simulink model "drawWorks_withLookup"  (R2018b)
settings: Solver=ode3  StartTime=0.0  StopTime=inf  RelTol=1e-3
PreLoadFcn:
  | addpath('CAD_Files');
  | warning('off','sm:sli:setup:compile:LocalSolverNotSupported');
  | 
  | loadScale = 3;
  | load limitsLookup.mat;
InitFcn:
  | Ts = 10e-4;        % SPS/Overall Simulation time step
  | Tssc = 10*Ts;       % Simscape simulation time step
  | 
  | G = 10;
  | Rdrum = 0.25;
  | Np = 5;
  | m_topdrive = 1000;
  | m_drillstring = 22500;
  | Rpulley = Rdrum;
  | 
  | m = m_topdrive + m_drillstring;
  | 
  | % Top/Bottom Distance
  | xtop = 48*0.3048;
  | xbott = 0;
  | 
  | % Maximum Torque/Power of Drive
  | Tmax = 8000*1.36;
  | Pmax = 1500*746;
  | 
  | % Initial Conditions
  | v0 = 0; %m/s
  | x0 = 0; %m
  | 
  | % Gravity
  | g = 9.8;
values from neighbouring files (symbols this model uses):
  distLowering = [-48 -47 -46 -45 -44 -43 -42 -41 -40 -39 -38 -37 ... (130 elements, 1x130)]    [limitsLookup.mat]
  distRaising = [0 0.1 0.2 0.3 0.4 0.5 0.6 0.7 0.8 0.9 1 1.1 ... (139 elements, 1x139)]    [limitsLookup.mat]
  loadIn = [23500 46000 68500 91000 93250 95500 97750 100000 102250 104500 106750 109000 ... (71 elements, 1x71)]    [DrawworksLimitData.mat]    (also in limitsLookup.mat)
  spdLowering = [-1500 -1500 -1500 -1500 -1500 -1500 -1500 -1500 -1500 -1500 -1483.12408278 -1433.71794393 ... (9230 elements, 71x130)]    [limitsLookup.mat]
  spdRaising = [7.42375457692 0 0 0 0 0 0 0 0 0 0 0 ... (9869 elements, 71x139)]    [limitsLookup.mat]
undefined symbols (not defined in the file or in its folder): DiscIntNeverNeededParam, X, Y, Z
libraries: sm_lib x38, fl_lib x14, nesl_utility x11, powerlib x6, simulink x6, spsDrivesDcBusModel x1
(part 1 of 2)
settings Model: Creator=jlesage  LastModifiedBy=jlesage
settings DataIOCC: SaveOutput=off  SignalLogging=off  DSMLogging=off  SaveTime=off
settings ExplorerConfigSet: InternalSimMechanicsExplorerSettings="<ExplorerConfiguration><canonicalview>default</canonicalview><AnimationSetting><BasePlaybackSpeed>1.0</BasePlaybackSpeed><PlaybackSpeedFactor>256.0</PlaybackSpeedFactor></AnimationSetting><TilePanel><TileInfo><Tiles Columns=\"1\" Count=\"1\" Rows=\"1\"><Column Weight=\"1\"/><Row Weight=\"1\"/><Tile Height=\"1\" Width=\"1\" X=\"0\" Y=\"0\"/></Tiles></TileInfo><SceneInfo><SceneViewer><BGColor><R>0.60000002384185791</R><G>0.60000002384185791</G><B>0.60000002384185791</B></BGColor><Camera><DoPerspective>off</DoPerspective><Position><X>4.3364080211050684</X><Y>-7.69010096822353528</Y><Z>10.5874852236011314</Z></Position><Center><X>-0.0853470869668693233</X><Y>1.05957776856095531</Y><Z>8.89555922243923014</Z></Center><Up><X>-0.0863591017029704255</X><Y>0.146899309055797511</Y><Z>0.985374395116894397</Z></Up><ViewLimDist>1</ViewLimDist><YLim>13.1346250998977876</YLim><XLim>16.5774012824701131</XLim></Camera></SceneViewer></SceneInfo></TilePanel><MechEditorPanel><Cameras/><GfxPanelCameraMap/><VideoCreator><PlaybackSpeedRatio>1.0</PlaybackSpeedRatio><FrameRate>30</FrameRate><VideoFormat>Motion JPEG AVI</VideoFormat><FrameSize>auto</FrameSize></VideoCreator></MechEditorPanel></ExplorerConfiguration>"

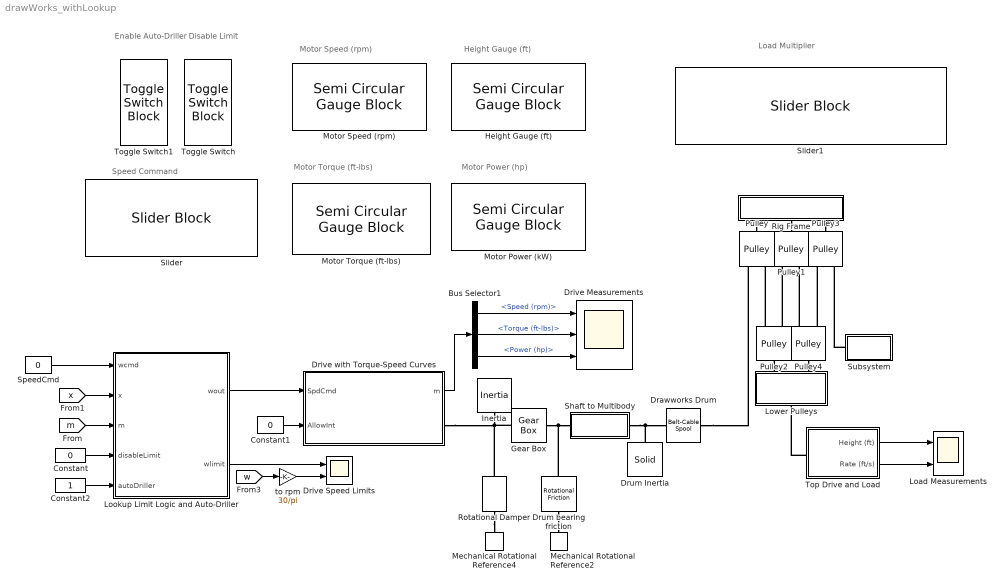
== system drawWorks_withLookup ==
  note: Height Gauge (ft)
  note: Motor Power (hp)
  note: Motor Torque (ft-lbs)
  note: Motor Speed (rpm)
  note: Load Multiplier
  note: Speed Command
  note: Disable
      | Limit
  note: Enable
      | Auto-Driller
  Bus Selector1 : BusSelector  OutputSignals=Mechanical.Speed (rpm),Mechanical.Torque (ft-lbs),Mechanical.Power (hp)
  Constant : Constant  Value=0  OutDataTypeStr=boolean
  Constant1 : Constant  Value=0
  Constant2 : Constant  OutDataTypeStr=boolean
  Drawworks Drum : sm_lib/Belts and Cables/Belt-Cable Spool  PitchRadius=Rdrum  PitchRadiusUnits=m  SenseSpoolAngleA=off  SenseFleetAngleA=off
      settings: SourceProductName=Simscape Multibody  SourceProductBaseCode=MS
  Drive Measurements : Scope  NumInputPorts=3
  Drive Speed Limits : Scope  NumInputPorts=2
  Drive with Torque-Speed Curves : Subsystem
  Drum Inertia : sm_lib/Body Elements/Solid  InertiaType=CalculateFromGeometry  Mass=0.01  MassUnits=kg  CenterOfMass=[0 0 0]  CenterOfMassUnits=m  MomentsOfInertia=[1 1 1]  MomentsOfInertiaUnits=kg*m^2  ProductsOfInertia=[0 0 0]  ProductsOfInertiaUnits=kg*m^2  BasedOnType=Density  Density=2700  DensityUnits=kg/m^3  DoExposeReferenceFrame=off  SerializedFrames=<Frames><Frame><Id>Frame1</Id><Value><Name>F1</Name><Origin><Source>ReferenceFrame</Source><FeatureName></FeatureName></Origin><PrimaryAxis><DefinedDirection>+Z</DefinedDirection><Source>ReferenceFrame</Source><SourceDirection>+Z</SourceDirection><FeatureName></FeatureName></PrimaryAxis><SecondaryAxis><DefinedDirection>+X</DefinedDirection><Source>ReferenceFrame</Source><SourceDirection>+X</SourceDirection><FeatureName></FeatureName></SecondaryAxis></Value></Frame></Frames>  GraphicType=FromGeometry  MarkerShape=Frame  MarkerSize=10  GraphicVisPropType=SimpleVisualProperties  GraphicDiffuseColor=[1.0 1.0 1.0]  GraphicSpecularColor=[0.8 0.8 0.8]  GraphicAmbientColor=[0.15 0.15 0.15 1.0]  GraphicEmissiveColor=[0.0 0.0 0.0 1.0]  GraphicShininess=10  GraphicOpacity=1.0  GeometryShape=Cylinder  RectangleSize=[1 1]  RectangleSizeUnits=m  BrickDimensions=[1 1 1]  BrickDimensionUnits=m  CylinderRadius=Rdrum  CylinderRadiusUnits=m  CylinderLength=0.75  CylinderLengthUnits=m  SphereRadius=0.5  SphereRadiusUnits=in  EllipsoidRadii=[1 1 1]*0.1  EllipsoidRadiiUnits=m  ExtrusionCrossSection=[1 1; -1 1; -1 -1; 1 -1]  ExtrusionCrossSectionUnits=m  ExtrusionLength=1  ExtrusionLengthUnits=m  PolygonNumSides=3  PolygonOuterRadius=1  PolygonOuterRadiusUnits=m  ExtGeomFileType=STEP  ExtGeomFileName=winch.step  ExtGeomFileUnits=m  RevolutionCrossSection=[1 1; 1 -1; 2 -1; 2 1]  RevolutionCrossSectionUnits=m  RevolutionExtent=Full  RevolutionAngle=180  RevolutionAngleUnits=deg
  Drum bearing friction : fl_lib/Mechanical/Rotational Elements/Rotational Friction  brkwy_trq=0.02*1.1 N*m  brkwy_vel=0.060623 rad/s  Col_trq=0.02 N*m  visc_coef=0.001 N*m/(rad/s)  w_specify=on  w_priority=Low  w=0 rad/s  w_nominal_specify=off  w_nominal_unit=rad/s  w_nominal_value=1  t_specify=off  t_priority=High  t=0 N*m  t_nominal_specify=off  t_nominal_unit=N*m  t_nominal_value=1
      settings: SourceProductName=Simscape
  Gear Box : fl_lib/Mechanical/Mechanisms/Gear Box  ratio=G  t_in_specify=off  t_in_priority=None  t_in=0 N*m  t_in_nominal_specify=off  t_in_nominal_unit=N*m  t_in_nominal_value=1  t_out_specify=off  t_out_priority=None  t_out=0 N*m  t_out_nominal_specify=off  t_out_nominal_unit=N*m  t_out_nominal_value=1
  Height Gauge (ft) : SemiCircularGaugeBlock  WebBlockId=1281  LabelPosition=Hide  ScaleMax=50  TickInterval=10
  Inertia : fl_lib/Mechanical/Rotational Elements/Inertia  inertia=0.01 kg*m^2  w_specify=off  w_priority=High  w=0 rad/s  w_nominal_specify=off  w_nominal_unit=rad/s  w_nominal_value=1  t_specify=off  t_priority=High  t=0 N*m  t_nominal_specify=off  t_nominal_unit=N*m  t_nominal_value=1
  Load Measurements : Scope  NumInputPorts=2
  Lookup Limit Logic and Auto-Driller : Stateflow chart  TreatAsAtomicUnit=on  SystemSampleTime=Tssc
  Lower Pulleys : Subsystem
  Mechanical Rotational Reference2 : fl_lib/Mechanical/Rotational Elements/Mechanical Rotational Reference
  Mechanical Rotational Reference4 : fl_lib/Mechanical/Rotational Elements/Mechanical Rotational Reference
  Motor Power (kW) : SemiCircularGaugeBlock  WebBlockId=1282  ScaleMin=-2000  ScaleMax=2000  TickInterval=1000
  Motor Speed (rpm) : SemiCircularGaugeBlock  WebBlockId=1283  ScaleMin=-1500  ScaleMax=1500  TickInterval=500
  Motor Torque (ft-lbs) : SemiCircularGaugeBlock  WebBlockId=1284  ScaleMin=-15000  ScaleMax=15000  TickInterval=5000
  Pulley{,1..4} (5 alike) : sm_lib/Belts and Cables/Pulley  PitchRadius=Rdrum  PitchRadiusUnits=m  SenseWrapAngle=off  SensePulleyAngleA=off  SensePulleyAngleB=off  SenseFleetAngleA=off  SenseFleetAngleB=off
      settings: SourceProductName=Simscape Multibody  SourceProductBaseCode=MS
  Rig Frame : Subsystem
  Rotational Damper : fl_lib/Mechanical/Rotational Elements/Rotational Damper  D=0.001 N*m/(rad/s)  w_specify=off  w_priority=High  w=0 rad/s  w_nominal_specify=off  w_nominal_unit=rad/s  w_nominal_value=1  t_specify=off  t_priority=High  t=0 N*m  t_nominal_specify=off  t_nominal_unit=N*m  t_nominal_value=1
  Shaft to Multibody : Subsystem
  Slider : SliderBlock  WebBlockId=1132  LabelPosition=Hide  ScaleMin=-1500  ScaleMax=1500
  Slider1 : SliderBlock  WebBlockId=1290  LabelPosition=Hide  ScaleMax=8  TickInterval=1
  SpeedCmd : Constant  Value=0  OutDataTypeStr=double
  Subsystem : Subsystem
  Toggle Switch : ToggleSwitchBlock  WebBlockId=1329  LabelPosition=Hide
      settings: Values={{'Off', 'On'}, [0 1]}
  Toggle Switch1 : ToggleSwitchBlock  WebBlockId=1330  LabelPosition=Hide
      settings: Values={{'Off', 'On'}, [0 1]}
  Top Drive and Load : Subsystem
  to rpm : Gain  Gain=30/pi
  wires:
  Bus Selector1/2 -> Drive Measurements/2  "<Torque (ft-lbs)>"
  Bus Selector1/3 -> Drive Measurements/3  "<Power (hp)>"
  Bus Selector1/1 -> Drive Measurements/1  "<Speed (rpm)>"
  [w] -> to rpm/1
  to rpm/1 -> Drive Speed Limits/2
  Constant1/1 -> Drive with Torque-Speed Curves/2(AllowInt)
  Drive with Torque-Speed Curves/1(m) -> Bus Selector1/1
  Top Drive and Load/1(Height (ft)) -> Load Measurements/1
  Top Drive and Load/2(Rate (ft/s)) -> Load Measurements/2
  SpeedCmd/1 -> Lookup Limit Logic and Auto-Driller/1(wcmd)
  [m] -> Lookup Limit Logic and Auto-Driller/3(m)
  [x] -> Lookup Limit Logic and Auto-Driller/2(x)
  Lookup Limit Logic and Auto-Driller/1(wout) -> Drive with Torque-Speed Curves/1(SpdCmd)
  Lookup Limit Logic and Auto-Driller/2(wlimit) -> Drive Speed Limits/1
  Constant2/1 -> Lookup Limit Logic and Auto-Driller/5(autoDriller)
  Constant/1 -> Lookup Limit Logic and Auto-Driller/4(disableLimit)
  connections:
  Drawworks Drum/RConn1 -- Pulley/RConn1
  Pulley4/RConn1 -- Pulley1/RConn2
  Pulley2/RConn1 -- Pulley/RConn2
  Subsystem/LConn1 -- Pulley3/RConn2
  Pulley4/RConn2 -- Pulley3/RConn1
  Pulley2/RConn2 -- Pulley1/RConn1
  Rig Frame/RConn1 -- Pulley/LConn1
  Rig Frame/RConn2 -- Pulley1/LConn1
  Rig Frame/RConn3 -- Pulley3/LConn1
  Lower Pulleys/RConn1 -- Pulley2/LConn1
  Pulley4/LConn1 -- Lower Pulleys/RConn2
  Drum Inertia/LConn1 -- Drawworks Drum/LConn1 -- Shaft to Multibody/RConn1
  Drum bearing friction/LConn1 -- Gear Box/RConn1 -- Shaft to Multibody/LConn1
  Drum bearing friction/RConn1 -- Mechanical Rotational Reference2/LConn1
  Rotational Damper/RConn1 -- Mechanical Rotational Reference4/LConn1
  Rotational Damper/LConn1 -- Gear Box/LConn1 -- Drive with Torque-Speed Curves/RConn1 -- Inertia/LConn1
  Top Drive and Load/LConn1 -- Lower Pulleys/LConn1

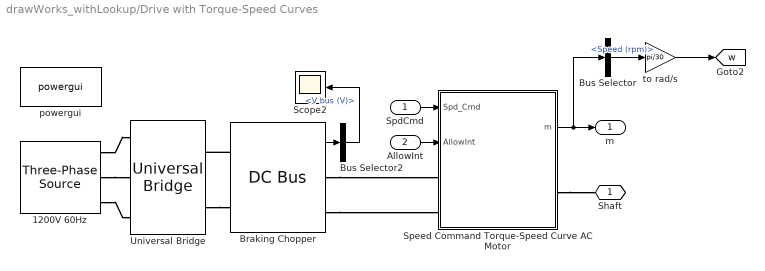
== system drawWorks_withLookup/Drive with Torque-Speed Curves ==
  SpdCmd : Inport
  AllowInt : Inport  Port=2
  1200V 60Hz : powerlib/Electrical Sources/Three-Phase Source  InternalConnection=Yg  VoltagePhases=off  Voltage=1200  PhaseAngle=0  Voltage_phases=[25e3 25e3 25e3]/sqrt(3)  PhaseAngles_phases=[0 -120 +120]  Frequency=60  NonIdealSource=off  SpecifyImpedance=on  Resistance=0.02  Inductance=0.05e-3  ShortCircuitLevel=500e6  BaseVoltage=5000  XRratio=7  BusType=swing  Pref=0  Qref=0  Prefabc=[10e3, 10e3, 10e3]  Qrefabc=[0, 0, 0]  Qmin=-inf  Qmax=inf
      settings: SourceProductName=Simscape Electrical
  Braking Chopper : spsDrivesDcBusModel/DC Bus   busType=Capacitive (generic)  Ts=Ts  capacitance=7500e-4  inductance=1e-3  Setx0=on  InitialVoltage=1000  Rbrake=8  frequency=500  activationVoltage=1200  shutdownVoltage=500
      settings: SourceProductName=The database C:\Users\ak23510\AppData\Roaming\MathWorks\MATLAB\R2017a\slblocks_master.db is locked, or a table in the database is locked. (database is locked)
  Bus Selector : BusSelector  OutputSignals=Mechanical.Speed (rpm)
  Bus Selector2 : BusSelector  OutputSignals=V bus (V)
  Scope2 : Scope
  Speed Command Torque-Speed Curve AC Motor : Subsystem  mask{contTrq=[10880,10880,10177,8905,7915,7124,6476,5699,4749,4071,3562], contSpd=[0 600 700 800 900 1000 1100 1250 1500 1750 2000], intTrq=[10880,10880,10177,8905,7915,7124,6476,5699,4749,4071,3562], intSpd=[0 600 700 800 900 1000 1100 1250 1500 1750 2000], intTime=1.5, offTime=7, Kp=15, Ki=1.5, wrate=750, Eff=99, T_alg=0.01}
      mask prompts: contTrq "Continuous Torque Limit (ft-lbs)"; contSpd "Continuous Speed Vector (rpm)"; intTrq "Intermittent Torque Limit (ft-lbs)"; intSpd "Intermittent Speed Vector (rpm)"; intTime "Time allowed above Steady-State (s)"; offTime "Cooldown Time (s)"; Kp "Speed Proportional Gain, Kp"; Ki "Speed Integral Gain, Ki"; wrate "Speed rate (rpm/s)"; Eff "Power Motor Efficiency (%)"; T_alg "Power Algebraic Loop Time Constant (s)"
      mask DialogControl Container4 Prompt: Torque-Speed Curves
      mask DialogControl Container6 Prompt: Controls
  Universal Bridge : powerlib/Power Electronics/Universal Bridge  Arms=3  SnubberResistance=1e5  SnubberCapacitance=inf  Device=Diodes  Ron=1e-3  Lon=0  ForwardVoltages="[  0  0  ]"  ForwardVoltage=0  GTOparameters=[ 10e-6 , 20e-6 ]  IGBTparameters=[ 1e-6 , 2e-6 ]  Measurements=All voltages and currents  Measurements_2=None  converterType=Rectifier
  powergui : powerlib/powergui  Priority=1  SimulationMode=Discrete  SampleTime=Ts  frequency=60  Iterations=50  frequencyindice=60  Pbase=100e6  ErrMax=1e-4  UnitsV=kV  UnitsW=MW  buscounter=0  FunctionMessages=off  echomessages=off  EnableUseOfTLC=off  CurrentSourceSwitches=off  DisableSnubberDevices=off  DisableRonSwitches=off  DisableVfSwitches=off  DisplayEquations=off  SolverType=Tustin/Backward Euler (TBE)  Interpol=off  ExternalGateDelay=off  methode=off  Ts=100  x0status=blocks  SPID=on  SwTol=0  HookPort=off  RestoreLinks=warning  ResistiveCurrentMeasurement=off  Frange=[0:2:500]  Ylog=off  Xlog=on  ShowGrid=off  save=off  variable=ZData  structure=0  ZoomFFT=off  StartTime=0.0  cycles=1  DisplayStyle=1  fundamental=60  FreqAxis=off  MaxFrequency=1000  frequencyindicesteady=1  RmsSteady=1  display=off
  to rad/s : Gain  Gain=pi/30
  Shaft : PMIOPort  Side=Right
  m : Outport
  tag scope: w=global
  wires:
  Braking Chopper/1 -> Bus Selector2/1
  Bus Selector2/1 -> Scope2/1  "<V bus (V)>"
  SpdCmd/1 -> Speed Command Torque-Speed Curve AC Motor/1(Spd_Cmd)
  AllowInt/1 -> Speed Command Torque-Speed Curve AC Motor/2(AllowInt)
  Speed Command Torque-Speed Curve AC Motor/1(m) -> Bus Selector/1, m/1
  to rad/s/1 -> [w]
  Bus Selector/1 -> to rad/s/1  "<Speed (rpm)>"
  connections:
  1200V 60Hz/RConn3 -- Universal Bridge/LConn3
  1200V 60Hz/RConn2 -- Universal Bridge/LConn2
  Braking Chopper/RConn2 -- Speed Command Torque-Speed Curve AC Motor/LConn2
  Braking Chopper/RConn1 -- Speed Command Torque-Speed Curve AC Motor/LConn1
  1200V 60Hz/RConn1 -- Universal Bridge/LConn1
  Braking Chopper/LConn1 -- Universal Bridge/RConn1
  Universal Bridge/RConn2 -- Braking Chopper/LConn2
  Speed Command Torque-Speed Curve AC Motor/RConn1 -- Shaft/RConn1

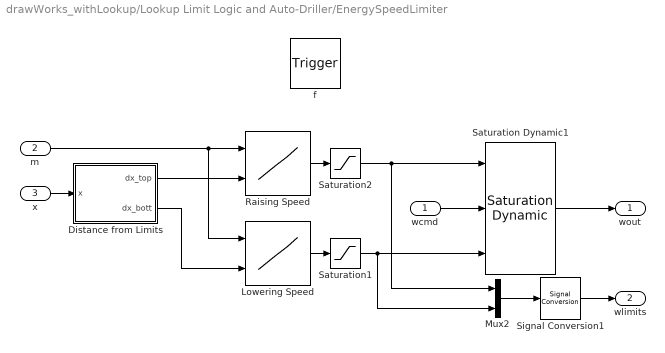
== system drawWorks_withLookup/Lookup Limit Logic and Auto-Driller/EnergySpeedLimiter ==
  wcmd : Inport  OutDataTypeStr=double  PortDimensions=1
  m : Inport  Port=2  OutDataTypeStr=double  PortDimensions=1
  x : Inport  Port=3  OutDataTypeStr=double  PortDimensions=1
  f : TriggerPort  TriggerType=function-call  VariantControl=(inherit)
      settings: CopyFcn=Stateflow.SLINSF.SimulinkMan.removeBlockPreDeleteFcn  PreDeleteFcn=Stateflow.SLINSF.SimulinkMan.unsafePredeleteFcn
  Distance from Limits : Subsystem
  Lowering Speed : Lookup_n-D  BreakpointsForDimension1=loadIn  BreakpointsForDimension2=distLowering  Table=spdLowering  InternalRulePriority=Speed  RndMeth=Simplest  InputSameDT=on
  Mux2 : Mux  Inputs=2
  Raising Speed : Lookup_n-D  BreakpointsForDimension1=loadIn  BreakpointsForDimension2=distRaising  Table=spdRaising  InternalRulePriority=Speed  RndMeth=Simplest  InputSameDT=on
  Saturation Dynamic1 : simulink/Discontinuities/Saturation Dynamic  OutMin=[]  OutMax=[]  OutDataTypeStr=Inherit: Same as second input  OutDataType=fixdt(1, 16)  OutScaling=2^-10  DoSatur=off
  Saturation1 : Saturate  UpperLimit=0  LowerLimit=-inf
  Saturation2 : Saturate  UpperLimit=inf  LowerLimit=0
  Signal Conversion1 : SignalConversion  OverrideOpt=off
  wout : Outport
  wlimits : Outport  Port=2
  wires:
  x/1 -> Distance from Limits/1(x)
  Saturation Dynamic1/1 -> wout/1
  Mux2/1 -> Signal Conversion1/1
  m/1 -> Lowering Speed/1, Raising Speed/1
  wcmd/1 -> Saturation Dynamic1/2
  Distance from Limits/2(dx_bott) -> Lowering Speed/2
  Distance from Limits/1(dx_top) -> Raising Speed/2
  Saturation1/1 -> Mux2/2, Saturation Dynamic1/3
  Lowering Speed/1 -> Saturation1/1
  Raising Speed/1 -> Saturation2/1
  Saturation2/1 -> Mux2/1, Saturation Dynamic1/1
  Signal Conversion1/1 -> wlimits/1

== system drawWorks_withLookup/Lower Pulleys ==
  Pulley 1 : Subsystem  mask{bottOffset=0.1}
      mask prompts: bottOffset "Bottom Offset"
  Pulley 2 : Subsystem  mask{bottOffset=-0.1}
      mask prompts: bottOffset "Bottom Offset"
  Load : PMIOPort  Side=Left
  P1 : PMIOPort  Port=2  Side=Right
  P2 : PMIOPort  Port=3  Side=Right
  connections:
  Pulley 1/LConn1 -- Pulley 2/LConn1 -- Load/RConn1
  Pulley 2/RConn1 -- P2/RConn1
  Pulley 1/RConn1 -- P1/RConn1

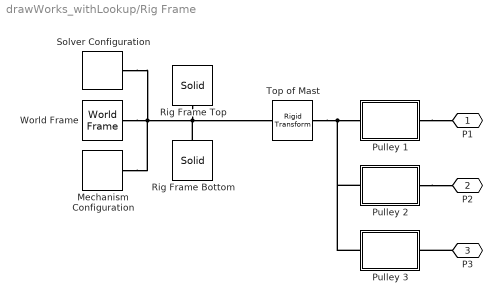
== system drawWorks_withLookup/Rig Frame ==
  Mechanism Configuration : sm_lib/Utilities/Mechanism Configuration  UniformGravity=Constant  GravityVector=[0 0 -9.80665]  GravityUnits=m/s^2  LinearizationDelta=0.001
  Pulley 1 : Subsystem  mask{topOffset=0.2}
      mask prompts: topOffset "Top Position [m]"
  Pulley 2 : Subsystem  mask{topOffset=0}
      mask prompts: topOffset "Top Position [m]"
  Pulley 3 : Subsystem  mask{topOffset=-0.2}
      mask prompts: topOffset "Top Position [m]"
  Rig Frame Top : sm_lib/Body Elements/Solid  InertiaType=CalculateFromGeometry  Mass=0.01  MassUnits=kg  CenterOfMass=[0 0 0]  CenterOfMassUnits=m  MomentsOfInertia=[1 1 1]  MomentsOfInertiaUnits=kg*m^2  ProductsOfInertia=[0 0 0]  ProductsOfInertiaUnits=kg*m^2  BasedOnType=Density  Density=2700  DensityUnits=kg/m^3  DoExposeReferenceFrame=off  SerializedFrames=<Frames><Frame><Id>Frame1</Id><Value><Name>F1</Name><Origin><Source>ReferenceFrame</Source><FeatureName></FeatureName></Origin><PrimaryAxis><DefinedDirection>+Z</DefinedDirection><Source>ReferenceFrame</Source><SourceDirection>+Y</SourceDirection><FeatureName></FeatureName></PrimaryAxis><SecondaryAxis><DefinedDirection>+X</DefinedDirection><Source>ReferenceFrame</Source><SourceDirection>+X</SourceDirection><FeatureName></FeatureName></SecondaryAxis></Value></Frame></Frames>  GraphicType=FromGeometry  MarkerShape=Frame  MarkerSize=10  GraphicVisPropType=SimpleVisualProperties  GraphicDiffuseColor=[1.0 0.0 0.2]  GraphicSpecularColor=[0.8 0.8 0.8]  GraphicAmbientColor=[0.15 0.15 0.15 1.0]  GraphicEmissiveColor=[0.0 0.0 0.0 1.0]  GraphicShininess=10  GraphicOpacity=1.0  GeometryShape=FromFile  RectangleSize=[1 1]  RectangleSizeUnits=m  BrickDimensions=[1 1 1]  BrickDimensionUnits=m  CylinderRadius=0.25  CylinderRadiusUnits=in  CylinderLength=1  CylinderLengthUnits=in  SphereRadius=0.5  SphereRadiusUnits=in  EllipsoidRadii=[1 1 1]*0.1  EllipsoidRadiiUnits=m  ExtrusionCrossSection=[1 1; -1 1; -1 -1; 1 -1]  ExtrusionCrossSectionUnits=m  ExtrusionLength=1  ExtrusionLengthUnits=m  PolygonNumSides=3  PolygonOuterRadius=1  PolygonOuterRadiusUnits=m  ExtGeomFileType=STEP  ExtGeomFileName=\CAD_Files\RigFrame_Top.STEP  ExtGeomFileUnits=m  RevolutionCrossSection=[1 1; 1 -1; 2 -1; 2 1]  RevolutionCrossSectionUnits=m  RevolutionExtent=Full  RevolutionAngle=180  RevolutionAngleUnits=deg
  Rig Frame Bottom : sm_lib/Body Elements/Solid  InertiaType=CalculateFromGeometry  Mass=0.01  MassUnits=kg  CenterOfMass=[0 0 0]  CenterOfMassUnits=m  MomentsOfInertia=[1 1 1]  MomentsOfInertiaUnits=kg*m^2  ProductsOfInertia=[0 0 0]  ProductsOfInertiaUnits=kg*m^2  BasedOnType=Density  Density=2700  DensityUnits=kg/m^3  DoExposeReferenceFrame=off  SerializedFrames=<Frames><Frame><Id>Frame1</Id><Value><Name>F1</Name><Origin><Source>ReferenceFrame</Source><FeatureName></FeatureName></Origin><PrimaryAxis><DefinedDirection>+Z</DefinedDirection><Source>ReferenceFrame</Source><SourceDirection>+Y</SourceDirection><FeatureName></FeatureName></PrimaryAxis><SecondaryAxis><DefinedDirection>+X</DefinedDirection><Source>ReferenceFrame</Source><SourceDirection>+X</SourceDirection><FeatureName></FeatureName></SecondaryAxis></Value></Frame></Frames>  GraphicType=FromGeometry  MarkerShape=Frame  MarkerSize=10  GraphicVisPropType=SimpleVisualProperties  GraphicDiffuseColor=[1.0 1.0 1.0]  GraphicSpecularColor=[0.8 0.8 0.8]  GraphicAmbientColor=[0.15 0.15 0.15 1.0]  GraphicEmissiveColor=[0.0 0.0 0.0 1.0]  GraphicShininess=10  GraphicOpacity=1.0  GeometryShape=FromFile  RectangleSize=[1 1]  RectangleSizeUnits=m  BrickDimensions=[1 1 1]  BrickDimensionUnits=m  CylinderRadius=0.25  CylinderRadiusUnits=in  CylinderLength=1  CylinderLengthUnits=in  SphereRadius=0.5  SphereRadiusUnits=in  EllipsoidRadii=[1 1 1]*0.1  EllipsoidRadiiUnits=m  ExtrusionCrossSection=[1 1; -1 1; -1 -1; 1 -1]  ExtrusionCrossSectionUnits=m  ExtrusionLength=1  ExtrusionLengthUnits=m  PolygonNumSides=3  PolygonOuterRadius=1  PolygonOuterRadiusUnits=m  ExtGeomFileType=STEP  ExtGeomFileName=\CAD_Files\RigFrame_Bottom.STEP  ExtGeomFileUnits=m  RevolutionCrossSection=[1 1; 1 -1; 2 -1; 2 1]  RevolutionCrossSectionUnits=m  RevolutionExtent=Full  RevolutionAngle=180  RevolutionAngleUnits=deg
  "Solver Configuration " : nesl_utility/Solver Configuration  PhysicalDomain=network_engine_domain  SubClassName=solver  LeftPortType=input  RightPortType=generic  Tones=[]  Harmonics=[]  SimulateNoise=off  Profile=off  UseLocalSampling=off  EnableSwitchedLinearOptims=on  FrequencyDomain=off  UseCCode=off  RelTol=0.001  AbsTol=1e-06  MinStep=1e-09  ToWorkspace=off  RevertToSquareIcSolve=off  NumHomotopyIterations=100  PhasorMode=off  PhasorModeNumHarmonics=1  DoDC=off  ResidualTolerance=1e-09  UseLocalSolver=on  LocalSolverChoice=NE_BACKWARD_EULER_ADVANCER  LocalSolverSampleTime=Tssc  DoFixedCost=on  MaxNonlinIter=3  MaxModeIter=2  LinearAlgebra=Sparse  EquationFormulation=NE_TIME_EF  DelaysMemoryBudget=1024  AutomaticFiltering=on  FilteringTimeConstant=0.001  PartitionStorageMethod=AS_NEEDED  PartitionMemoryBudget=1024
  Top of Mast : sm_lib/Frames and Transforms/Rigid Transform  TranslationMethod=Cartesian  TranslationStandardOffset=57.5  TranslationLengthUnit=ft  TranslationStandardAxis=+Z  TranslationCartesianOffset=[0 0 57.5]  TranslationROffset=0  TranslationROffsetUnits=m  TranslationZOffset=0  TranslationZOffsetUnits=m  TranslationThetaOffset=0  TranslationThetaOffsetUnits=deg  RotationMethod=StandardAxis  RotationAngleUnits=deg  RotationStandardAxis=+Y  RotationAngle=90  RotationArbitraryAxis=[0 0 1]  FollAlignAxisA=+X  BaseAlignAxisA=+Y  FollAlignAxisB=+Y  BaseAlignAxisB=+Z  RotationSequenceAxes=FollowerAxes  RotationSequence=XYX  RotationSequenceAngles=[0 0 0]  RotationSequenceAnglesUnits=deg  RotationMatrix=[1 0 0; 0 1 0; 0 0 1]
  World Frame : sm_lib/Frames and Transforms/World Frame
  P1 : PMIOPort  Side=Right
  P2 : PMIOPort  Port=2  Side=Right
  P3 : PMIOPort  Port=3  Side=Right
  connections:
  Top of Mast/RConn1 -- Pulley 3/LConn1 -- Pulley 2/LConn1 -- Pulley 1/LConn1
  Mechanism Configuration/RConn1 -- "Solver Configuration "/RConn1 -- World Frame/RConn1 -- Top of Mast/LConn1 -- Rig Frame Top/LConn1 -- Rig Frame Bottom/LConn1
  Pulley 1/RConn1 -- P1/RConn1
  P3/RConn1 -- Pulley 3/RConn1
  Pulley 2/RConn1 -- P2/RConn1

== system drawWorks_withLookup/Shaft to Multibody ==
  Drum Position : sm_lib/Frames and Transforms/Rigid Transform  TranslationMethod=Cartesian  TranslationStandardOffset=10  TranslationLengthUnit=ft  TranslationStandardAxis=+Y  TranslationCartesianOffset=[5 10 0]  TranslationROffset=0  TranslationROffsetUnits=m  TranslationZOffset=0  TranslationZOffsetUnits=m  TranslationThetaOffset=0  TranslationThetaOffsetUnits=deg  RotationMethod=StandardAxis  RotationAngleUnits=deg  RotationStandardAxis=-Y  RotationAngle=90  RotationArbitraryAxis=[0 0 1]  FollAlignAxisA=+X  BaseAlignAxisA=+Y  FollAlignAxisB=+Y  BaseAlignAxisB=+Z  RotationSequenceAxes=FollowerAxes  RotationSequence=XYX  RotationSequenceAngles=[0 0 0]  RotationSequenceAnglesUnits=deg  RotationMatrix=[1 0 0; 0 1 0; 0 0 1]
  Revolute Joint for Drum : sm_lib/Joints/Revolute Joint  SenseConstraintForce=off  SenseConstraintForceX=off  SenseConstraintForceY=off  SenseConstraintForceZ=off  SenseConstraintTorque=off  SenseConstraintTorqueX=off  SenseConstraintTorqueY=off  SenseConstraintTorqueZ=off  SenseTotalForce=off  SenseTotalForceX=off  SenseTotalForceY=off  SenseTotalForceZ=off  SenseTotalTorque=off  SenseTotalTorqueX=off  SenseTotalTorqueY=off  SenseTotalTorqueZ=off  CompositeWrenchDir=FollowerOnBase  CompositeWrenchFrame=BaseFrame  EquilibriumPosition=0  EquilibriumPositionUnits=deg  SpringStiffness=0  SpringStiffnessUnits=N*m/deg  DampingCoefficient=0  DampingCoefficientUnits=N*m/(deg/s)  TorqueActuationMode=InputTorque  MotionActuationMode=ComputedMotion  SensePosition=off  SenseVelocity=on  SenseAcceleration=off  SenseTorqueForce=off  PositionTargetSpecify=off  PositionTargetPriority=High  PositionTargetValue=0  PositionTargetValueUnits=deg  VelocityTargetSpecify=off  VelocityTargetPriority=High  VelocityTargetValue=0  VelocityTargetValueUnits=deg/s
  Rotational Simscape Intf : Subsystem
  World Frame2 : sm_lib/Frames and Transforms/World Frame
  Drum : PMIOPort  Side=Right
  Shaft : PMIOPort  Port=2  Side=Left
  connections:
  Drum Position/RConn1 -- Revolute Joint for Drum/LConn1
  Revolute Joint for Drum/RConn1 -- Drum/RConn1
  Rotational Simscape Intf/RConn1 -- Revolute Joint for Drum/LConn2
  World Frame2/RConn1 -- Drum Position/LConn1
  Shaft/RConn1 -- Rotational Simscape Intf/RConn2
  Rotational Simscape Intf/LConn1 -- Revolute Joint for Drum/RConn2

== system drawWorks_withLookup/Subsystem ==
  Anchor Position : sm_lib/Frames and Transforms/Rigid Transform  TranslationMethod=Cartesian  TranslationStandardOffset=10  TranslationLengthUnit=ft  TranslationStandardAxis=+Y  TranslationCartesianOffset=[-5 10+Rdrum*3.2808 0]  TranslationROffset=0  TranslationROffsetUnits=m  TranslationZOffset=0  TranslationZOffsetUnits=m  TranslationThetaOffset=0  TranslationThetaOffsetUnits=deg  RotationMethod=StandardAxis  RotationAngleUnits=deg  RotationStandardAxis=-Y  RotationAngle=90  RotationArbitraryAxis=[0 0 1]  FollAlignAxisA=+X  BaseAlignAxisA=+Y  FollAlignAxisB=+Y  BaseAlignAxisB=+Z  RotationSequenceAxes=FollowerAxes  RotationSequence=XYX  RotationSequenceAngles=[0 0 0]  RotationSequenceAnglesUnits=deg  RotationMatrix=[1 0 0; 0 1 0; 0 0 1]
  Belt-Cable Properties : sm_lib/Belts and Cables/Belt-Cable Properties  DrumBeltCableAlignment=Unrestricted  GraphicType=PitchLine  GraphicVisPropType=SimpleVisualProperties  GraphicDiffuseColor=[0.0 0.0 0.0]  GraphicSpecularColor=[0.5 0.5 0.5 1.0]  GraphicAmbientColor=[0.15 0.15 0.15 1.0]  GraphicEmissiveColor=[0.0 0.0 0.0 1.0]  GraphicShininess=75  GraphicOpacity=1.0
      settings: SourceProductName=Simscape Multibody  SourceProductBaseCode=MS
  Belt-Cable End : sm_lib/Belts and Cables/Belt-Cable End
      settings: SourceProductName=Simscape Multibody  SourceProductBaseCode=MS
  World Frame3 : sm_lib/Frames and Transforms/World Frame
  Anchor : PMIOPort  Side=Left
  connections:
  World Frame3/RConn1 -- Anchor Position/LConn1
  Anchor Position/RConn1 -- Belt-Cable End/LConn1
  Belt-Cable End/RConn1 -- Anchor/RConn1 -- Belt-Cable Properties/LConn1

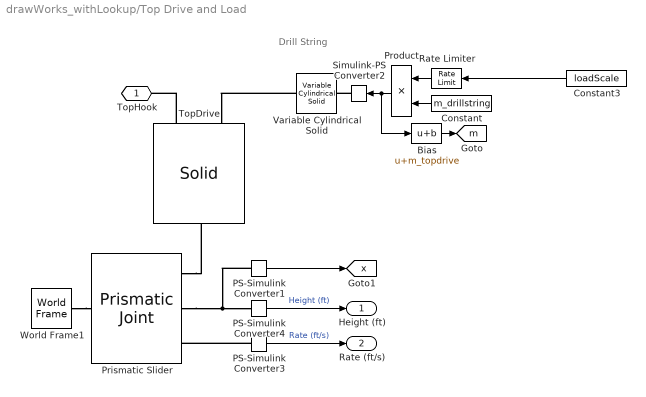
== system drawWorks_withLookup/Top Drive and Load ==
  note: Drill String
  Bias : Bias  Bias=m_topdrive
  Constant : Constant  Value=m_drillstring
  Constant3 : Constant  Value=loadScale
  PS-Simulink Converter1 : nesl_utility/PS-Simulink Converter  PhysicalDomain=network_engine_domain  SubClassName=ps_output  LeftPortType=input  RightPortType=output  PseudoPeriodic=off  Frequencies=[]  Unit=ft  AffineConversion=off
  PS-Simulink Converter3 : nesl_utility/PS-Simulink Converter  PhysicalDomain=network_engine_domain  SubClassName=ps_output  LeftPortType=input  RightPortType=output  PseudoPeriodic=off  Frequencies=[]  Unit=ft/s  AffineConversion=off
  PS-Simulink Converter4 : nesl_utility/PS-Simulink Converter  PhysicalDomain=network_engine_domain  SubClassName=ps_output  LeftPortType=input  RightPortType=output  PseudoPeriodic=off  Frequencies=[]  Unit=ft  AffineConversion=off
  Prismatic Slider : sm_lib/Joints/Prismatic Joint  SenseConstraintForce=off  SenseConstraintForceX=off  SenseConstraintForceY=off  SenseConstraintForceZ=off  SenseConstraintTorque=off  SenseConstraintTorqueX=off  SenseConstraintTorqueY=off  SenseConstraintTorqueZ=off  SenseTotalForce=off  SenseTotalForceX=off  SenseTotalForceY=off  SenseTotalForceZ=off  SenseTotalTorque=off  SenseTotalTorqueX=off  SenseTotalTorqueY=off  SenseTotalTorqueZ=off  CompositeWrenchDir=FollowerOnBase  CompositeWrenchFrame=BaseFrame  EquilibriumPosition=0  EquilibriumPositionUnits=m  SpringStiffness=0  SpringStiffnessUnits=N/m  DampingCoefficient=0  DampingCoefficientUnits=N/(m/s)  TorqueActuationMode=NoTorque  MotionActuationMode=ComputedMotion  SensePosition=on  SenseVelocity=on  SenseAcceleration=off  SenseTorqueForce=off  PositionTargetSpecify=off  PositionTargetPriority=High  PositionTargetValue=5  PositionTargetValueUnits=ft  VelocityTargetSpecify=off  VelocityTargetPriority=High  VelocityTargetValue=0  VelocityTargetValueUnits=m/s
  Product : Product
  Rate Limiter : RateLimiter  RisingSlewLimit=0.5  FallingSlewLimit=-0.5  SampleTimeMode=inherited  InitialCondition=loadScale
  Simulink-PS Converter2 : nesl_utility/Simulink-PS Converter  PhysicalDomain=network_engine_domain  SubClassName=ps_input  LeftPortType=input  RightPortType=output  PseudoPeriodic=off  Frequencies=[]  NoiseDistribution=none  NoiseParameters=[]  Unit=kg  AffineConversion=off  FilteringAndDerivatives=provide  SimscapeFilterOrder=1  InputFilterTimeConstant=0.001  UdotUserProvided=0
  TopDrive : sm_lib/Body Elements/Solid  InertiaType=PointMass  Mass=m_topdrive  MassUnits=kg  CenterOfMass=[0 0 0]  CenterOfMassUnits=m  MomentsOfInertia=[1 1 1]  MomentsOfInertiaUnits=kg*m^2  ProductsOfInertia=[0 0 0]  ProductsOfInertiaUnits=kg*m^2  BasedOnType=Density  Density=1000  DensityUnits=kg/m^3  DoExposeReferenceFrame=off  SerializedFrames=<Frames><Frame><Id>Frame1</Id><Value><Name>TopHook</Name><Origin><Source>GeometricFeature</Source><FeatureName>cylindrical surface 11</FeatureName></Origin><PrimaryAxis><DefinedDirection>+Z</DefinedDirection><Source>ReferenceFrame</Source><SourceDirection>+Y</SourceDirection><FeatureName></FeatureName></PrimaryAxis><SecondaryAxis><DefinedDirection>+X</DefinedDirection><Source>ReferenceFrame</Source><SourceDirection>+X</SourceDirection><FeatureName></FeatureName></SecondaryAxis></Value></Frame><Frame><Id>Frame2</Id><Value><Name>COM</Name><Origin><Source>GeometricFeature</Source><FeatureName>planar surface 22</FeatureName></Origin><PrimaryAxis><DefinedDirection>+Z</DefinedDirection><Source>ReferenceFrame</Source><SourceDirection>+Y</SourceDirection><FeatureName></FeatureName></PrimaryAxis><SecondaryAxis><DefinedDirection>+X</DefinedDirection><Source>ReferenceFrame</Source><SourceDirection>+X</SourceDirection><FeatureName></FeatureName></SecondaryAxis></Value></Frame><Frame><Id>Frame3</Id><Value><Name>String</Name><Origin><Source>GeometricFeature</Source><FeatureName>planar surface 23</FeatureName></Origin><PrimaryAxis><DefinedDirection>+Z</DefinedDirection><Source>ReferenceFrame</Source><SourceDirection>-Y</SourceDirection><FeatureName></FeatureName></PrimaryAxis><SecondaryAxis><DefinedDirection>+X</DefinedDirection><Source>ReferenceFrame</Source><SourceDirection>+X</SourceDirection><FeatureName></FeatureName></SecondaryAxis></Value></Frame></Frames>  GraphicType=FromGeometry  MarkerShape=Sphere  MarkerSize=10  GraphicVisPropType=SimpleVisualProperties  GraphicDiffuseColor=[0.8 0.8 0.0]  GraphicSpecularColor=[0.5 0.5 0.5 1.0]  GraphicAmbientColor=[0.15 0.15 0.15 1.0]  GraphicEmissiveColor=[0.0 0.0 0.0 1.0]  GraphicShininess=75  GraphicOpacity=1.0  GeometryShape=FromFile  RectangleSize=[1 1]  RectangleSizeUnits=m  BrickDimensions=[1 1 1]*4  BrickDimensionUnits=in  CylinderRadius=1  CylinderRadiusUnits=m  CylinderLength=1  CylinderLengthUnits=m  SphereRadius=1  SphereRadiusUnits=m  EllipsoidRadii=[1 1 1]  EllipsoidRadiiUnits=m  ExtrusionCrossSection=[1 1; -1 1; -1 -1; 1 -1]  ExtrusionCrossSectionUnits=m  ExtrusionLength=1  ExtrusionLengthUnits=m  PolygonNumSides=3  PolygonOuterRadius=1  PolygonOuterRadiusUnits=m  ExtGeomFileType=STEP  ExtGeomFileName=\CAD_Files\TopDrive.STEP  ExtGeomFileUnits=m  RevolutionCrossSection=[1 1; 1 -1; 2 -1; 2 1]  RevolutionCrossSectionUnits=m  RevolutionExtent=Full  RevolutionAngle=180  RevolutionAngleUnits=deg
  Variable Cylindrical Solid : sm_lib/Body Elements/Variable Mass/Variable Cylindrical Solid  LengthType=CalculateFromMass  Length=1  LengthUnits=m  RadiusType=Constant  Radius=0.1  RadiusUnits=m  MassType=ProvidedByInput  InitialMassType=Specified  InitialMass=1  InitialMassUnits=kg  Density=1000  DensityUnits=kg/m^3  SenseRadius=off  SenseLength=off  SenseMass=off  SenseCenterOfMass=off  SenseInertiaMatrix=off  GraphicType=Marker  MarkerShape=Cube  MarkerSize=10  GraphicVisPropType=SimpleVisualProperties  GraphicDiffuseColor=[0.5 0.5 0.5]  GraphicSpecularColor=[0.5 0.5 0.5 1.0]  GraphicAmbientColor=[0.15 0.15 0.15 1.0]  GraphicEmissiveColor=[0.0 0.0 0.0 1.0]  GraphicShininess=75  GraphicOpacity=1.0
      settings: SourceProductName=Simscape Multibody  SourceProductBaseCode=MS
  World Frame1 : sm_lib/Frames and Transforms/World Frame
  TopHook : PMIOPort  Side=Left
  Height (ft) : Outport
  Rate (ft/s) : Outport  Port=2
  tag scope: m=global, x=global
  wires:
  PS-Simulink Converter1/1 -> [x]
  Constant/1 -> Product/2
  Bias/1 -> [m]
  Constant3/1 -> Rate Limiter/1
  Product/1 -> Bias/1, Simulink-PS Converter2/1
  PS-Simulink Converter4/1 -> Height (ft)/1  "Height (ft)"
  PS-Simulink Converter3/1 -> Rate (ft/s)/1  "Rate (ft/s)"
  Rate Limiter/1 -> Product/1
  connections:
  Prismatic Slider/RConn2 -- PS-Simulink Converter1/LConn1 -- PS-Simulink Converter4/LConn1
  Prismatic Slider/RConn1 -- TopDrive/RConn1
  Simulink-PS Converter2/RConn1 -- Variable Cylindrical Solid/LConn1
  Variable Cylindrical Solid/RConn1 -- TopDrive/LConn2
  World Frame1/RConn1 -- Prismatic Slider/LConn1
  PS-Simulink Converter3/LConn1 -- Prismatic Slider/RConn3
  TopDrive/LConn1 -- TopHook/RConn1

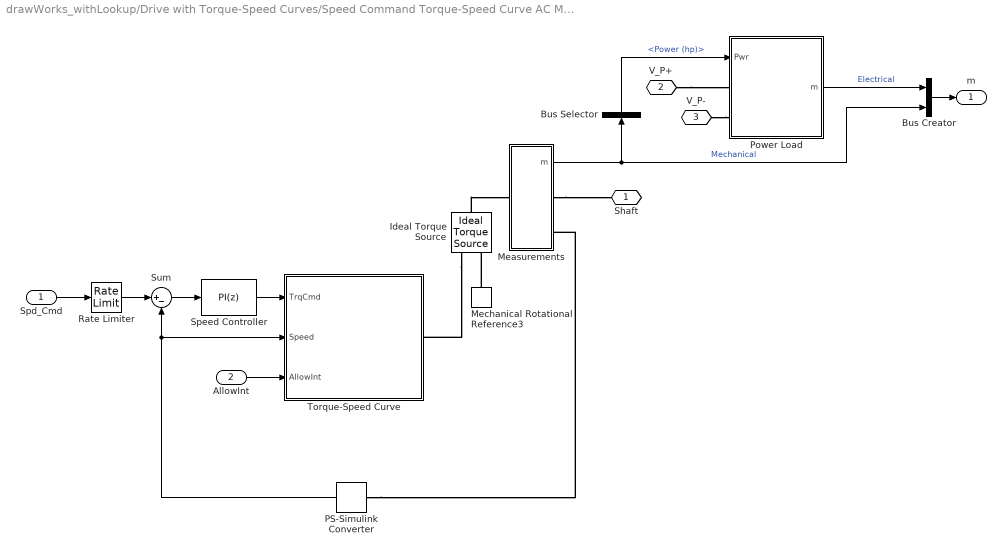
== system drawWorks_withLookup/Drive with Torque-Speed Curves/Speed Command Torque-Speed Curve AC Motor ==
  Spd_Cmd : Inport
  AllowInt : Inport  Port=2
  Bus Creator : BusCreator  Inputs=2
  Bus Selector : BusSelector  OutputSignals=Power (hp)
  Ideal Torque Source : fl_lib/Mechanical/Mechanical Sources/Ideal Torque Source
  Measurements : Subsystem
  Mechanical Rotational Reference3 : fl_lib/Mechanical/Rotational Elements/Mechanical Rotational Reference
  PS-Simulink Converter : nesl_utility/PS-Simulink Converter  PhysicalDomain=network_engine_domain  SubClassName=ps_output  LeftPortType=input  RightPortType=output  PseudoPeriodic=off  Frequencies=[]  Unit=rpm  AffineConversion=off
  Power Load : Subsystem  VariantControl=Variant
  Rate Limiter : RateLimiter  RisingSlewLimit=wrate  FallingSlewLimit=-wrate  SampleTimeMode=inherited
  Speed Controller : simulink/Continuous/PID Controller  Controller=PI  Form=Parallel  TimeDomain=Discrete-time  SampleTime=-1  IntegratorMethod=Forward Euler  FilterMethod=Forward Euler  ControllerParametersSource=internal  P=Kp  I=Ki  D=-9.19425038888835  UseFilter=on  N=3.08252405545653  TunerSelectOption=Transfer Function Based (PID Tuner App)  ZeroCross=off  InitialConditionSource=internal  InitialConditionForIntegrator=Rdrum/(G*(Np-1))*(m_topdrive+m_drillstring)*9.81*0.737562*loadScale  InitialConditionForFilter=0  DifferentiatorICPrevScaledInput=0  ExternalReset=none  TrackingMode=off  Kt=1  LimitOutput=on  UpperSaturationLimit=intTrq(1)  LowerSaturationLimit=-intTrq(1)  LinearizeAsGain=on  AntiWindupMode=clamping  Kb=1000  POutMin=[]  POutMax=[]  IOutMin=[]  IOutMax=[]  DOutMin=[]  DOutMax=[]  NOutMin=[]  NOutMax=[]  SumOutMin=[]  SumOutMax=[]  SaturationOutMin=[]  SaturationOutMax=[]  PParamMin=[]  PParamMax=[]  IParamMin=[]  IParamMax=[]  DParamMin=[]  DParamMax=[]  NParamMin=[]  NParamMax=[]  KbParamMin=[]  KbParamMax=[]  KtParamMin=[]  KtParamMax=[]  KbOutMin=[]  KbOutMax=[]  KtOutMin=[]  KtOutMax=[]  IntegratorOutMin=[]  IntegratorOutMax=[]  FilterOutMin=[]  FilterOutMax=[]  SumI1OutMin=[]  SumI1OutMax=[]  SumI2OutMin=[]  SumI2OutMax=[]  SumI3OutMin=[]  SumI3OutMax=[]  SumI4OutMin=[]  SumI4OutMax=[]  SumDOutMin=[]  SumDOutMax=[]  DifferentiatorOutMin=[]  DifferentiatorOutMax=[]  FilterDiffOutCoefMin=[]  FilterDiffOutCoefMax=[]  ReciprocalOutMin=[]  ReciprocalOutMax=[]  SumDenOutMin=[]  SumDenOutMax=[]  SumNumOutMin=[]  SumNumOutMax=[]  DivideOutMin=[]  DivideOutMax=[]  IntegratorContinuousStateAttributes=''  IntegratorStateMustResolveToSignalObject=off  IntegratorRTWStateStorageClass=Auto  FilterContinuousStateAttributes=''  FilterStateMustResolveToSignalObject=off  FilterRTWStateStorageClass=Auto  ParallelPVariant=InternalParameters  IdealPVariant=Disabled  IVariant=InternalParameters  DVariant=Disabled  IntegratorVariant=Discrete  SatVariant=Enabled  AWVariant=DiscClampingParallel  PCopyVariant=Disabled  TRVariant=Disabled  FdbkBlocksVariant=Forward  IdealPFdbkVariant=Disabled  SatFdbkVariant=Disabled  DerivativeFilterVariant=Disabled  NVariant=Disabled  NCopyVariant=Disabled_SignalSpec  FilterICVariant=Disabled  IntegratorICVariant=InternalICs  ExternalResetVariant=Disabled  TRSumVariant=Passthrough  SumFdbkVariant=Disabled  SumVariant=Sum_PI
  Sum : Sum  Inputs=|+-
  Torque-Speed Curve : Subsystem
  Shaft : PMIOPort  Side=Right
  V_P+ : PMIOPort  Port=2  Side=Left
  V_P- : PMIOPort  Port=3  Side=Left
  m : Outport
  wires:
  Measurements/1(m) -> Bus Selector/1, Bus Creator/2  "Mechanical"
  Rate Limiter/1 -> Sum/1
  Sum/1 -> Speed Controller/1
  Speed Controller/1 -> Torque-Speed Curve/1(TrqCmd)
  AllowInt/1 -> Torque-Speed Curve/3(AllowInt)
  PS-Simulink Converter/1 -> Sum/2, Torque-Speed Curve/2(Speed)
  Spd_Cmd/1 -> Rate Limiter/1
  Bus Selector/1 -> Power Load/1(Pwr)  "<Power (hp)>"
  Bus Creator/1 -> m/1
  Power Load/1(m) -> Bus Creator/1  "Electrical"
  connections:
  Mechanical Rotational Reference3/LConn1 -- Ideal Torque Source/RConn2
  Ideal Torque Source/LConn1 -- Measurements/LConn1
  PS-Simulink Converter/LConn1 -- Measurements/RConn2
  Measurements/RConn1 -- Shaft/RConn1
  Ideal Torque Source/RConn1 -- Torque-Speed Curve/RConn1
  V_P-/RConn1 -- Power Load/LConn2
  V_P+/RConn1 -- Power Load/LConn1

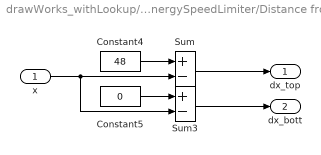
== system drawWorks_withLookup/Lookup Limit Logic and Auto-Driller/EnergySpeedLimiter/Distance from Limits ==
  x : Inport
  Constant4 : Constant  Value=48
  Constant5 : Constant  Value=0
  Sum : Sum  Inputs=+-
  Sum3 : Sum  Inputs=+-
  dx_top : Outport
  dx_bott : Outport  Port=2
  wires:
  Constant4/1 -> Sum/1
  Constant5/1 -> Sum3/1
  x/1 -> Sum/2, Sum3/2
  Sum/1 -> dx_top/1
  Sum3/1 -> dx_bott/1

== system drawWorks_withLookup/Lower Pulleys/Pulley 1 ==
  Offset from Load : sm_lib/Frames and Transforms/Rigid Transform  TranslationMethod=Cartesian  TranslationStandardOffset=57.5  TranslationLengthUnit=m  TranslationStandardAxis=+Z  TranslationCartesianOffset=[bottOffset 0 0]  TranslationROffset=0  TranslationROffsetUnits=m  TranslationZOffset=0  TranslationZOffsetUnits=m  TranslationThetaOffset=0  TranslationThetaOffsetUnits=deg  RotationMethod=StandardAxis  RotationAngleUnits=deg  RotationStandardAxis=+Y  RotationAngle=90  RotationArbitraryAxis=[0 0 1]  FollAlignAxisA=+X  BaseAlignAxisA=+Y  FollAlignAxisB=+Y  BaseAlignAxisB=+Z  RotationSequenceAxes=FollowerAxes  RotationSequence=XYX  RotationSequenceAngles=[0 0 0]  RotationSequenceAnglesUnits=deg  RotationMatrix=[1 0 0; 0 1 0; 0 0 1]
  Pulley Inertia : sm_lib/Body Elements/Solid  InertiaType=CalculateFromGeometry  Mass=0.01  MassUnits=kg  CenterOfMass=[0 0 0]  CenterOfMassUnits=m  MomentsOfInertia=[1 1 1]  MomentsOfInertiaUnits=kg*m^2  ProductsOfInertia=[0 0 0]  ProductsOfInertiaUnits=kg*m^2  BasedOnType=Density  Density=2700  DensityUnits=kg/m^3  DoExposeReferenceFrame=off  SerializedFrames=<Frames><Frame><Id>Frame1</Id><Value><Name>F1</Name><Origin><Source>GeometricFeature</Source><FeatureName>top surface</FeatureName></Origin><PrimaryAxis><DefinedDirection>+Z</DefinedDirection><Source>ReferenceFrame</Source><SourceDirection>+Z</SourceDirection><FeatureName></FeatureName></PrimaryAxis><SecondaryAxis><DefinedDirection>+X</DefinedDirection><Source>ReferenceFrame</Source><SourceDirection>+X</SourceDirection><FeatureName></FeatureName></SecondaryAxis></Value></Frame></Frames>  GraphicType=FromGeometry  MarkerShape=Frame  MarkerSize=10  GraphicVisPropType=SimpleVisualProperties  GraphicDiffuseColor=[1.0 1.0 1.0]  GraphicSpecularColor=[0.8 0.8 0.8]  GraphicAmbientColor=[0.15 0.15 0.15 1.0]  GraphicEmissiveColor=[0.0 0.0 0.0 1.0]  GraphicShininess=10  GraphicOpacity=1.0  GeometryShape=Cylinder  RectangleSize=[1 1]  RectangleSizeUnits=m  BrickDimensions=[1 1 1]  BrickDimensionUnits=m  CylinderRadius=Rpulley  CylinderRadiusUnits=m  CylinderLength=2  CylinderLengthUnits=in  SphereRadius=0.5  SphereRadiusUnits=in  EllipsoidRadii=[1 1 1]*0.1  EllipsoidRadiiUnits=m  ExtrusionCrossSection=[1 1; -1 1; -1 -1; 1 -1]  ExtrusionCrossSectionUnits=m  ExtrusionLength=1  ExtrusionLengthUnits=m  PolygonNumSides=3  PolygonOuterRadius=1  PolygonOuterRadiusUnits=m  ExtGeomFileType=STEP  ExtGeomFileName=winch.step  ExtGeomFileUnits=m  RevolutionCrossSection=[1 1; 1 -1; 2 -1; 2 1]  RevolutionCrossSectionUnits=m  RevolutionExtent=Full  RevolutionAngle=180  RevolutionAngleUnits=deg
  Revolute Joint : sm_lib/Joints/Revolute Joint  SenseConstraintForce=off  SenseConstraintForceX=off  SenseConstraintForceY=off  SenseConstraintForceZ=off  SenseConstraintTorque=off  SenseConstraintTorqueX=off  SenseConstraintTorqueY=off  SenseConstraintTorqueZ=off  SenseTotalForce=off  SenseTotalForceX=off  SenseTotalForceY=off  SenseTotalForceZ=off  SenseTotalTorque=off  SenseTotalTorqueX=off  SenseTotalTorqueY=off  SenseTotalTorqueZ=off  CompositeWrenchDir=FollowerOnBase  CompositeWrenchFrame=BaseFrame  EquilibriumPosition=0  EquilibriumPositionUnits=deg  SpringStiffness=0  SpringStiffnessUnits=N*m/deg  DampingCoefficient=0  DampingCoefficientUnits=N*m/(deg/s)  TorqueActuationMode=NoTorque  MotionActuationMode=ComputedMotion  SensePosition=off  SenseVelocity=off  SenseAcceleration=off  SenseTorqueForce=off  PositionTargetSpecify=off  PositionTargetPriority=High  PositionTargetValue=0  PositionTargetValueUnits=deg  VelocityTargetSpecify=off  VelocityTargetPriority=High  VelocityTargetValue=0  VelocityTargetValueUnits=deg/s
  Load : PMIOPort  Side=Left
  Pulley : PMIOPort  Port=2  Side=Right
  connections:
  Offset from Load/LConn1 -- Load/RConn1
  Pulley Inertia/LConn1 -- Pulley/RConn1 -- Revolute Joint/RConn1
  Offset from Load/RConn1 -- Revolute Joint/LConn1

== system drawWorks_withLookup/Lower Pulleys/Pulley 2 ==
  Offset from Load : sm_lib/Frames and Transforms/Rigid Transform  TranslationMethod=Cartesian  TranslationStandardOffset=57.5  TranslationLengthUnit=m  TranslationStandardAxis=+Z  TranslationCartesianOffset=[bottOffset 0 0]  TranslationROffset=0  TranslationROffsetUnits=m  TranslationZOffset=0  TranslationZOffsetUnits=m  TranslationThetaOffset=0  TranslationThetaOffsetUnits=deg  RotationMethod=StandardAxis  RotationAngleUnits=deg  RotationStandardAxis=+Y  RotationAngle=90  RotationArbitraryAxis=[0 0 1]  FollAlignAxisA=+X  BaseAlignAxisA=+Y  FollAlignAxisB=+Y  BaseAlignAxisB=+Z  RotationSequenceAxes=FollowerAxes  RotationSequence=XYX  RotationSequenceAngles=[0 0 0]  RotationSequenceAnglesUnits=deg  RotationMatrix=[1 0 0; 0 1 0; 0 0 1]
  Pulley Inertia : sm_lib/Body Elements/Solid  InertiaType=CalculateFromGeometry  Mass=0.01  MassUnits=kg  CenterOfMass=[0 0 0]  CenterOfMassUnits=m  MomentsOfInertia=[1 1 1]  MomentsOfInertiaUnits=kg*m^2  ProductsOfInertia=[0 0 0]  ProductsOfInertiaUnits=kg*m^2  BasedOnType=Density  Density=2700  DensityUnits=kg/m^3  DoExposeReferenceFrame=off  SerializedFrames=<Frames><Frame><Id>Frame1</Id><Value><Name>F1</Name><Origin><Source>GeometricFeature</Source><FeatureName>top surface</FeatureName></Origin><PrimaryAxis><DefinedDirection>+Z</DefinedDirection><Source>ReferenceFrame</Source><SourceDirection>+Z</SourceDirection><FeatureName></FeatureName></PrimaryAxis><SecondaryAxis><DefinedDirection>+X</DefinedDirection><Source>ReferenceFrame</Source><SourceDirection>+X</SourceDirection><FeatureName></FeatureName></SecondaryAxis></Value></Frame></Frames>  GraphicType=FromGeometry  MarkerShape=Frame  MarkerSize=10  GraphicVisPropType=SimpleVisualProperties  GraphicDiffuseColor=[1.0 1.0 1.0]  GraphicSpecularColor=[0.8 0.8 0.8]  GraphicAmbientColor=[0.15 0.15 0.15 1.0]  GraphicEmissiveColor=[0.0 0.0 0.0 1.0]  GraphicShininess=10  GraphicOpacity=1.0  GeometryShape=Cylinder  RectangleSize=[1 1]  RectangleSizeUnits=m  BrickDimensions=[1 1 1]  BrickDimensionUnits=m  CylinderRadius=Rpulley  CylinderRadiusUnits=m  CylinderLength=2  CylinderLengthUnits=in  SphereRadius=0.5  SphereRadiusUnits=in  EllipsoidRadii=[1 1 1]*0.1  EllipsoidRadiiUnits=m  ExtrusionCrossSection=[1 1; -1 1; -1 -1; 1 -1]  ExtrusionCrossSectionUnits=m  ExtrusionLength=1  ExtrusionLengthUnits=m  PolygonNumSides=3  PolygonOuterRadius=1  PolygonOuterRadiusUnits=m  ExtGeomFileType=STEP  ExtGeomFileName=winch.step  ExtGeomFileUnits=m  RevolutionCrossSection=[1 1; 1 -1; 2 -1; 2 1]  RevolutionCrossSectionUnits=m  RevolutionExtent=Full  RevolutionAngle=180  RevolutionAngleUnits=deg
  Revolute Joint : sm_lib/Joints/Revolute Joint  SenseConstraintForce=off  SenseConstraintForceX=off  SenseConstraintForceY=off  SenseConstraintForceZ=off  SenseConstraintTorque=off  SenseConstraintTorqueX=off  SenseConstraintTorqueY=off  SenseConstraintTorqueZ=off  SenseTotalForce=off  SenseTotalForceX=off  SenseTotalForceY=off  SenseTotalForceZ=off  SenseTotalTorque=off  SenseTotalTorqueX=off  SenseTotalTorqueY=off  SenseTotalTorqueZ=off  CompositeWrenchDir=FollowerOnBase  CompositeWrenchFrame=BaseFrame  EquilibriumPosition=0  EquilibriumPositionUnits=deg  SpringStiffness=0  SpringStiffnessUnits=N*m/deg  DampingCoefficient=0  DampingCoefficientUnits=N*m/(deg/s)  TorqueActuationMode=NoTorque  MotionActuationMode=ComputedMotion  SensePosition=off  SenseVelocity=off  SenseAcceleration=off  SenseTorqueForce=off  PositionTargetSpecify=off  PositionTargetPriority=High  PositionTargetValue=0  PositionTargetValueUnits=deg  VelocityTargetSpecify=off  VelocityTargetPriority=High  VelocityTargetValue=0  VelocityTargetValueUnits=deg/s
  Load : PMIOPort  Side=Left
  Pulley : PMIOPort  Port=2  Side=Right
  connections:
  Offset from Load/LConn1 -- Load/RConn1
  Revolute Joint/RConn1 -- Pulley Inertia/LConn1 -- Pulley/RConn1
  Offset from Load/RConn1 -- Revolute Joint/LConn1
